simulink model "rx2"  (R2022b)
settings: Solver=FixedStepDiscrete  StartTime=0.0  StopTime=3.3E6  FixedStep=1  RelTol=1e-3  EnableMultiTasking=on
model workspace (MAT data in the model file):
  mwTaskManagerKernelLatency = 0
undefined symbols (not defined in the file or in its folder): Add, jsin, magnitude, rom_pilot_conj_tt, Shift
libraries: hdlsllib x3231, whdlutilities x525, simulink x260, whdlmod x112, whdledac x26, dsphdlmathfun2 x24, commchan3 x1
(part 50 of 59)

== system rx2/process3/decoder/p-p/Subsystem2/Subsystem/Subsystem1/Subsystem/Subsystem4 ==
  data2 : Inport  OutDataTypeStr=data_type
  wr_addr1 : Inport  Port=2
  wr_en2 : Inport  Port=3
  rd_addr1 : Inport  Port=4
  Mux1 : Mux  Inputs=2
  Selector : Selector  InputPortWidth=4  IndexOptions=Index vector (dialog)  Indices=[1:2]  OutputSizes=1
  Selector1 : Selector  InputPortWidth=4  IndexOptions=Index vector (dialog)  Indices=[3:4]  OutputSizes=1
  Subsystem : Subsystem
  Subsystem1 : Subsystem
  rd_dout1 : Outport  PortDimensions=4  VectorParamsAs1DForOutWhenUnconnected=off
  wires:
  Selector/1 -> Subsystem/1(data)
  Subsystem/1(rd_dout) -> Mux1/1
  Subsystem1/1(rd_dout) -> Mux1/2
  wr_addr1/1 -> Subsystem/2(wr_addr), Subsystem1/2(wr_addr)
  Selector1/1 -> Subsystem1/1(data)
  wr_en2/1 -> Subsystem/3(wr_en), Subsystem1/3(wr_en)
  data2/1 -> Selector1/1, Selector/1
  Mux1/1 -> rd_dout1/1
  rd_addr1/1 -> Subsystem/4(rd_addr), Subsystem1/4(rd_addr)

== system rx2/process3/decoder/p-p/Subsystem2/Subsystem/Subsystem1/Subsystem1/Subsystem1 ==
  data2 : Inport  OutDataTypeStr=data_type
  wr_addr1 : Inport  Port=2
  wr_en2 : Inport  Port=3
  rd_addr1 : Inport  Port=4
  Mux1 : Mux  Inputs=2
  Selector : Selector  InputPortWidth=4  IndexOptions=Index vector (dialog)  Indices=[1:2]  OutputSizes=1
  Selector1 : Selector  InputPortWidth=4  IndexOptions=Index vector (dialog)  Indices=[3:4]  OutputSizes=1
  Subsystem : Subsystem
  Subsystem1 : Subsystem
  rd_dout1 : Outport  PortDimensions=4  VectorParamsAs1DForOutWhenUnconnected=off
  wires:
  rd_addr1/1 -> Subsystem1/4(rd_addr), Subsystem/4(rd_addr)
  Mux1/1 -> rd_dout1/1
  data2/1 -> Selector/1, Selector1/1
  wr_en2/1 -> Subsystem1/3(wr_en), Subsystem/3(wr_en)
  Selector1/1 -> Subsystem1/1(data)
  wr_addr1/1 -> Subsystem1/2(wr_addr), Subsystem/2(wr_addr)
  Subsystem1/1(rd_dout) -> Mux1/2
  Subsystem/1(rd_dout) -> Mux1/1
  Selector/1 -> Subsystem/1(data)

== system rx2/process3/decoder/p-p/Subsystem2/Subsystem/Subsystem1/Subsystem1/Subsystem4 ==
  data2 : Inport  OutDataTypeStr=data_type
  wr_addr1 : Inport  Port=2
  wr_en2 : Inport  Port=3
  rd_addr1 : Inport  Port=4
  Mux1 : Mux  Inputs=2
  Selector : Selector  InputPortWidth=4  IndexOptions=Index vector (dialog)  Indices=[1:2]  OutputSizes=1
  Selector1 : Selector  InputPortWidth=4  IndexOptions=Index vector (dialog)  Indices=[3:4]  OutputSizes=1
  Subsystem : Subsystem
  Subsystem1 : Subsystem
  rd_dout1 : Outport  PortDimensions=4  VectorParamsAs1DForOutWhenUnconnected=off
  wires:
  rd_addr1/1 -> Subsystem1/4(rd_addr), Subsystem/4(rd_addr)
  Mux1/1 -> rd_dout1/1
  data2/1 -> Selector/1, Selector1/1
  wr_en2/1 -> Subsystem1/3(wr_en), Subsystem/3(wr_en)
  Selector1/1 -> Subsystem1/1(data)
  wr_addr1/1 -> Subsystem1/2(wr_addr), Subsystem/2(wr_addr)
  Subsystem1/1(rd_dout) -> Mux1/2
  Subsystem/1(rd_dout) -> Mux1/1
  Selector/1 -> Subsystem/1(data)

== system rx2/process3/decoder/p-p/Subsystem2/Subsystem/Subsystem2/Subsystem/Subsystem1 ==
  data2 : Inport  OutDataTypeStr=data_type
  wr_addr1 : Inport  Port=2
  wr_en2 : Inport  Port=3
  rd_addr1 : Inport  Port=4
  Mux1 : Mux  Inputs=2
  Selector : Selector  InputPortWidth=4  IndexOptions=Index vector (dialog)  Indices=[1:2]  OutputSizes=1
  Selector1 : Selector  InputPortWidth=4  IndexOptions=Index vector (dialog)  Indices=[3:4]  OutputSizes=1
  Subsystem : Subsystem
  Subsystem1 : Subsystem
  rd_dout1 : Outport  PortDimensions=4  VectorParamsAs1DForOutWhenUnconnected=off
  wires:
  rd_addr1/1 -> Subsystem1/4(rd_addr), Subsystem/4(rd_addr)
  Mux1/1 -> rd_dout1/1
  data2/1 -> Selector/1, Selector1/1
  wr_en2/1 -> Subsystem1/3(wr_en), Subsystem/3(wr_en)
  Selector1/1 -> Subsystem1/1(data)
  wr_addr1/1 -> Subsystem1/2(wr_addr), Subsystem/2(wr_addr)
  Subsystem1/1(rd_dout) -> Mux1/2
  Subsystem/1(rd_dout) -> Mux1/1
  Selector/1 -> Subsystem/1(data)

== system rx2/process3/decoder/p-p/Subsystem2/Subsystem/Subsystem2/Subsystem/Subsystem4 ==
  data2 : Inport  OutDataTypeStr=data_type
  wr_addr1 : Inport  Port=2
  wr_en2 : Inport  Port=3
  rd_addr1 : Inport  Port=4
  Mux1 : Mux  Inputs=2
  Selector : Selector  InputPortWidth=4  IndexOptions=Index vector (dialog)  Indices=[1:2]  OutputSizes=1
  Selector1 : Selector  InputPortWidth=4  IndexOptions=Index vector (dialog)  Indices=[3:4]  OutputSizes=1
  Subsystem : Subsystem
  Subsystem1 : Subsystem
  rd_dout1 : Outport  PortDimensions=4  VectorParamsAs1DForOutWhenUnconnected=off
  wires:
  Selector/1 -> Subsystem/1(data)
  Subsystem/1(rd_dout) -> Mux1/1
  Subsystem1/1(rd_dout) -> Mux1/2
  wr_addr1/1 -> Subsystem/2(wr_addr), Subsystem1/2(wr_addr)
  Selector1/1 -> Subsystem1/1(data)
  wr_en2/1 -> Subsystem/3(wr_en), Subsystem1/3(wr_en)
  data2/1 -> Selector1/1, Selector/1
  Mux1/1 -> rd_dout1/1
  rd_addr1/1 -> Subsystem/4(rd_addr), Subsystem1/4(rd_addr)

== system rx2/process3/decoder/p-p/Subsystem2/Subsystem/Subsystem2/Subsystem1/Subsystem1 ==
  data2 : Inport  OutDataTypeStr=data_type
  wr_addr1 : Inport  Port=2
  wr_en2 : Inport  Port=3
  rd_addr1 : Inport  Port=4
  Mux1 : Mux  Inputs=2
  Selector : Selector  InputPortWidth=4  IndexOptions=Index vector (dialog)  Indices=[1:2]  OutputSizes=1
  Selector1 : Selector  InputPortWidth=4  IndexOptions=Index vector (dialog)  Indices=[3:4]  OutputSizes=1
  Subsystem : Subsystem
  Subsystem1 : Subsystem
  rd_dout1 : Outport  PortDimensions=4  VectorParamsAs1DForOutWhenUnconnected=off
  wires:
  rd_addr1/1 -> Subsystem1/4(rd_addr), Subsystem/4(rd_addr)
  Mux1/1 -> rd_dout1/1
  data2/1 -> Selector/1, Selector1/1
  wr_en2/1 -> Subsystem1/3(wr_en), Subsystem/3(wr_en)
  Selector1/1 -> Subsystem1/1(data)
  wr_addr1/1 -> Subsystem1/2(wr_addr), Subsystem/2(wr_addr)
  Subsystem1/1(rd_dout) -> Mux1/2
  Subsystem/1(rd_dout) -> Mux1/1
  Selector/1 -> Subsystem/1(data)

== system rx2/process3/decoder/p-p/Subsystem2/Subsystem/Subsystem2/Subsystem1/Subsystem4 ==
  data2 : Inport  OutDataTypeStr=data_type
  wr_addr1 : Inport  Port=2
  wr_en2 : Inport  Port=3
  rd_addr1 : Inport  Port=4
  Mux1 : Mux  Inputs=2
  Selector : Selector  InputPortWidth=4  IndexOptions=Index vector (dialog)  Indices=[1:2]  OutputSizes=1
  Selector1 : Selector  InputPortWidth=4  IndexOptions=Index vector (dialog)  Indices=[3:4]  OutputSizes=1
  Subsystem : Subsystem
  Subsystem1 : Subsystem
  rd_dout1 : Outport  PortDimensions=4  VectorParamsAs1DForOutWhenUnconnected=off
  wires:
  rd_addr1/1 -> Subsystem1/4(rd_addr), Subsystem/4(rd_addr)
  Mux1/1 -> rd_dout1/1
  data2/1 -> Selector/1, Selector1/1
  wr_en2/1 -> Subsystem1/3(wr_en), Subsystem/3(wr_en)
  Selector1/1 -> Subsystem1/1(data)
  wr_addr1/1 -> Subsystem1/2(wr_addr), Subsystem/2(wr_addr)
  Subsystem1/1(rd_dout) -> Mux1/2
  Subsystem/1(rd_dout) -> Mux1/1
  Selector/1 -> Subsystem/1(data)

== system rx2/process3/decoder/p-p/Subsystem2/Subsystem1/Subsystem1/Subsystem/Subsystem1 ==
  data2 : Inport  OutDataTypeStr=data_type
  wr_addr1 : Inport  Port=2
  wr_en2 : Inport  Port=3
  rd_addr1 : Inport  Port=4
  Mux1 : Mux  Inputs=2
  Selector : Selector  InputPortWidth=4  IndexOptions=Index vector (dialog)  Indices=[1:2]  OutputSizes=1
  Selector1 : Selector  InputPortWidth=4  IndexOptions=Index vector (dialog)  Indices=[3:4]  OutputSizes=1
  Subsystem : Subsystem
  Subsystem1 : Subsystem
  rd_dout1 : Outport  PortDimensions=4  VectorParamsAs1DForOutWhenUnconnected=off
  wires:
  rd_addr1/1 -> Subsystem1/4(rd_addr), Subsystem/4(rd_addr)
  Mux1/1 -> rd_dout1/1
  data2/1 -> Selector/1, Selector1/1
  wr_en2/1 -> Subsystem1/3(wr_en), Subsystem/3(wr_en)
  Selector1/1 -> Subsystem1/1(data)
  wr_addr1/1 -> Subsystem1/2(wr_addr), Subsystem/2(wr_addr)
  Subsystem1/1(rd_dout) -> Mux1/2
  Subsystem/1(rd_dout) -> Mux1/1
  Selector/1 -> Subsystem/1(data)

== system rx2/process3/decoder/p-p/Subsystem2/Subsystem1/Subsystem1/Subsystem/Subsystem4 ==
  data2 : Inport  OutDataTypeStr=data_type
  wr_addr1 : Inport  Port=2
  wr_en2 : Inport  Port=3
  rd_addr1 : Inport  Port=4
  Mux1 : Mux  Inputs=2
  Selector : Selector  InputPortWidth=4  IndexOptions=Index vector (dialog)  Indices=[1:2]  OutputSizes=1
  Selector1 : Selector  InputPortWidth=4  IndexOptions=Index vector (dialog)  Indices=[3:4]  OutputSizes=1
  Subsystem : Subsystem
  Subsystem1 : Subsystem
  rd_dout1 : Outport  PortDimensions=4  VectorParamsAs1DForOutWhenUnconnected=off
  wires:
  Selector/1 -> Subsystem/1(data)
  Subsystem/1(rd_dout) -> Mux1/1
  Subsystem1/1(rd_dout) -> Mux1/2
  wr_addr1/1 -> Subsystem/2(wr_addr), Subsystem1/2(wr_addr)
  Selector1/1 -> Subsystem1/1(data)
  wr_en2/1 -> Subsystem/3(wr_en), Subsystem1/3(wr_en)
  data2/1 -> Selector1/1, Selector/1
  Mux1/1 -> rd_dout1/1
  rd_addr1/1 -> Subsystem/4(rd_addr), Subsystem1/4(rd_addr)

== system rx2/process3/decoder/p-p/Subsystem2/Subsystem1/Subsystem1/Subsystem1/Subsystem1 ==
  data2 : Inport  OutDataTypeStr=data_type
  wr_addr1 : Inport  Port=2
  wr_en2 : Inport  Port=3
  rd_addr1 : Inport  Port=4
  Mux1 : Mux  Inputs=2
  Selector : Selector  InputPortWidth=4  IndexOptions=Index vector (dialog)  Indices=[1:2]  OutputSizes=1
  Selector1 : Selector  InputPortWidth=4  IndexOptions=Index vector (dialog)  Indices=[3:4]  OutputSizes=1
  Subsystem : Subsystem
  Subsystem1 : Subsystem
  rd_dout1 : Outport  PortDimensions=4  VectorParamsAs1DForOutWhenUnconnected=off
  wires:
  rd_addr1/1 -> Subsystem1/4(rd_addr), Subsystem/4(rd_addr)
  Mux1/1 -> rd_dout1/1
  data2/1 -> Selector/1, Selector1/1
  wr_en2/1 -> Subsystem1/3(wr_en), Subsystem/3(wr_en)
  Selector1/1 -> Subsystem1/1(data)
  wr_addr1/1 -> Subsystem1/2(wr_addr), Subsystem/2(wr_addr)
  Subsystem1/1(rd_dout) -> Mux1/2
  Subsystem/1(rd_dout) -> Mux1/1
  Selector/1 -> Subsystem/1(data)

== system rx2/process3/decoder/p-p/Subsystem2/Subsystem1/Subsystem1/Subsystem1/Subsystem4 ==
  data2 : Inport  OutDataTypeStr=data_type
  wr_addr1 : Inport  Port=2
  wr_en2 : Inport  Port=3
  rd_addr1 : Inport  Port=4
  Mux1 : Mux  Inputs=2
  Selector : Selector  InputPortWidth=4  IndexOptions=Index vector (dialog)  Indices=[1:2]  OutputSizes=1
  Selector1 : Selector  InputPortWidth=4  IndexOptions=Index vector (dialog)  Indices=[3:4]  OutputSizes=1
  Subsystem : Subsystem
  Subsystem1 : Subsystem
  rd_dout1 : Outport  PortDimensions=4  VectorParamsAs1DForOutWhenUnconnected=off
  wires:
  rd_addr1/1 -> Subsystem1/4(rd_addr), Subsystem/4(rd_addr)
  Mux1/1 -> rd_dout1/1
  data2/1 -> Selector/1, Selector1/1
  wr_en2/1 -> Subsystem1/3(wr_en), Subsystem/3(wr_en)
  Selector1/1 -> Subsystem1/1(data)
  wr_addr1/1 -> Subsystem1/2(wr_addr), Subsystem/2(wr_addr)
  Subsystem1/1(rd_dout) -> Mux1/2
  Subsystem/1(rd_dout) -> Mux1/1
  Selector/1 -> Subsystem/1(data)

== system rx2/process3/decoder/p-p/Subsystem2/Subsystem1/Subsystem2/Subsystem/Subsystem1 ==
  data2 : Inport  OutDataTypeStr=data_type
  wr_addr1 : Inport  Port=2
  wr_en2 : Inport  Port=3
  rd_addr1 : Inport  Port=4
  Mux1 : Mux  Inputs=2
  Selector : Selector  InputPortWidth=4  IndexOptions=Index vector (dialog)  Indices=[1:2]  OutputSizes=1
  Selector1 : Selector  InputPortWidth=4  IndexOptions=Index vector (dialog)  Indices=[3:4]  OutputSizes=1
  Subsystem : Subsystem
  Subsystem1 : Subsystem
  rd_dout1 : Outport  PortDimensions=4  VectorParamsAs1DForOutWhenUnconnected=off
  wires:
  rd_addr1/1 -> Subsystem1/4(rd_addr), Subsystem/4(rd_addr)
  Mux1/1 -> rd_dout1/1
  data2/1 -> Selector/1, Selector1/1
  wr_en2/1 -> Subsystem1/3(wr_en), Subsystem/3(wr_en)
  Selector1/1 -> Subsystem1/1(data)
  wr_addr1/1 -> Subsystem1/2(wr_addr), Subsystem/2(wr_addr)
  Subsystem1/1(rd_dout) -> Mux1/2
  Subsystem/1(rd_dout) -> Mux1/1
  Selector/1 -> Subsystem/1(data)

== system rx2/process3/decoder/p-p/Subsystem2/Subsystem1/Subsystem2/Subsystem/Subsystem4 ==
  data2 : Inport  OutDataTypeStr=data_type
  wr_addr1 : Inport  Port=2
  wr_en2 : Inport  Port=3
  rd_addr1 : Inport  Port=4
  Mux1 : Mux  Inputs=2
  Selector : Selector  InputPortWidth=4  IndexOptions=Index vector (dialog)  Indices=[1:2]  OutputSizes=1
  Selector1 : Selector  InputPortWidth=4  IndexOptions=Index vector (dialog)  Indices=[3:4]  OutputSizes=1
  Subsystem : Subsystem
  Subsystem1 : Subsystem
  rd_dout1 : Outport  PortDimensions=4  VectorParamsAs1DForOutWhenUnconnected=off
  wires:
  Selector/1 -> Subsystem/1(data)
  Subsystem/1(rd_dout) -> Mux1/1
  Subsystem1/1(rd_dout) -> Mux1/2
  wr_addr1/1 -> Subsystem/2(wr_addr), Subsystem1/2(wr_addr)
  Selector1/1 -> Subsystem1/1(data)
  wr_en2/1 -> Subsystem/3(wr_en), Subsystem1/3(wr_en)
  data2/1 -> Selector1/1, Selector/1
  Mux1/1 -> rd_dout1/1
  rd_addr1/1 -> Subsystem/4(rd_addr), Subsystem1/4(rd_addr)

== system rx2/process3/decoder/p-p/Subsystem2/Subsystem1/Subsystem2/Subsystem1/Subsystem1 ==
  data2 : Inport  OutDataTypeStr=data_type
  wr_addr1 : Inport  Port=2
  wr_en2 : Inport  Port=3
  rd_addr1 : Inport  Port=4
  Mux1 : Mux  Inputs=2
  Selector : Selector  InputPortWidth=4  IndexOptions=Index vector (dialog)  Indices=[1:2]  OutputSizes=1
  Selector1 : Selector  InputPortWidth=4  IndexOptions=Index vector (dialog)  Indices=[3:4]  OutputSizes=1
  Subsystem : Subsystem
  Subsystem1 : Subsystem
  rd_dout1 : Outport  PortDimensions=4  VectorParamsAs1DForOutWhenUnconnected=off
  wires:
  rd_addr1/1 -> Subsystem1/4(rd_addr), Subsystem/4(rd_addr)
  Mux1/1 -> rd_dout1/1
  data2/1 -> Selector/1, Selector1/1
  wr_en2/1 -> Subsystem1/3(wr_en), Subsystem/3(wr_en)
  Selector1/1 -> Subsystem1/1(data)
  wr_addr1/1 -> Subsystem1/2(wr_addr), Subsystem/2(wr_addr)
  Subsystem1/1(rd_dout) -> Mux1/2
  Subsystem/1(rd_dout) -> Mux1/1
  Selector/1 -> Subsystem/1(data)

== system rx2/process3/decoder/p-p/Subsystem2/Subsystem1/Subsystem2/Subsystem1/Subsystem4 ==
  data2 : Inport  OutDataTypeStr=data_type
  wr_addr1 : Inport  Port=2
  wr_en2 : Inport  Port=3
  rd_addr1 : Inport  Port=4
  Mux1 : Mux  Inputs=2
  Selector : Selector  InputPortWidth=4  IndexOptions=Index vector (dialog)  Indices=[1:2]  OutputSizes=1
  Selector1 : Selector  InputPortWidth=4  IndexOptions=Index vector (dialog)  Indices=[3:4]  OutputSizes=1
  Subsystem : Subsystem
  Subsystem1 : Subsystem
  rd_dout1 : Outport  PortDimensions=4  VectorParamsAs1DForOutWhenUnconnected=off
  wires:
  rd_addr1/1 -> Subsystem1/4(rd_addr), Subsystem/4(rd_addr)
  Mux1/1 -> rd_dout1/1
  data2/1 -> Selector/1, Selector1/1
  wr_en2/1 -> Subsystem1/3(wr_en), Subsystem/3(wr_en)
  Selector1/1 -> Subsystem1/1(data)
  wr_addr1/1 -> Subsystem1/2(wr_addr), Subsystem/2(wr_addr)
  Subsystem1/1(rd_dout) -> Mux1/2
  Subsystem/1(rd_dout) -> Mux1/1
  Selector/1 -> Subsystem/1(data)

== system rx2/process4/decoder/p-p/Subsystem2/Subsystem/Subsystem1/Subsystem/Subsystem1 ==
  data2 : Inport  OutDataTypeStr=data_type
  wr_addr1 : Inport  Port=2
  wr_en2 : Inport  Port=3
  rd_addr1 : Inport  Port=4
  Mux1 : Mux  Inputs=2
  Selector : Selector  InputPortWidth=4  IndexOptions=Index vector (dialog)  Indices=[1:2]  OutputSizes=1
  Selector1 : Selector  InputPortWidth=4  IndexOptions=Index vector (dialog)  Indices=[3:4]  OutputSizes=1
  Subsystem : Subsystem
  Subsystem1 : Subsystem
  rd_dout1 : Outport  PortDimensions=4  VectorParamsAs1DForOutWhenUnconnected=off
  wires:
  Selector/1 -> Subsystem/1(data)
  Subsystem/1(rd_dout) -> Mux1/1
  Subsystem1/1(rd_dout) -> Mux1/2
  wr_addr1/1 -> Subsystem/2(wr_addr), Subsystem1/2(wr_addr)
  Selector1/1 -> Subsystem1/1(data)
  wr_en2/1 -> Subsystem/3(wr_en), Subsystem1/3(wr_en)
  data2/1 -> Selector1/1, Selector/1
  Mux1/1 -> rd_dout1/1
  rd_addr1/1 -> Subsystem/4(rd_addr), Subsystem1/4(rd_addr)

== system rx2/process4/decoder/p-p/Subsystem2/Subsystem/Subsystem1/Subsystem/Subsystem4 ==
  data2 : Inport  OutDataTypeStr=data_type
  wr_addr1 : Inport  Port=2
  wr_en2 : Inport  Port=3
  rd_addr1 : Inport  Port=4
  Mux1 : Mux  Inputs=2
  Selector : Selector  InputPortWidth=4  IndexOptions=Index vector (dialog)  Indices=[1:2]  OutputSizes=1
  Selector1 : Selector  InputPortWidth=4  IndexOptions=Index vector (dialog)  Indices=[3:4]  OutputSizes=1
  Subsystem : Subsystem
  Subsystem1 : Subsystem
  rd_dout1 : Outport  PortDimensions=4  VectorParamsAs1DForOutWhenUnconnected=off
  wires:
  rd_addr1/1 -> Subsystem1/4(rd_addr), Subsystem/4(rd_addr)
  Mux1/1 -> rd_dout1/1
  data2/1 -> Selector/1, Selector1/1
  wr_en2/1 -> Subsystem1/3(wr_en), Subsystem/3(wr_en)
  Selector1/1 -> Subsystem1/1(data)
  wr_addr1/1 -> Subsystem1/2(wr_addr), Subsystem/2(wr_addr)
  Subsystem1/1(rd_dout) -> Mux1/2
  Subsystem/1(rd_dout) -> Mux1/1
  Selector/1 -> Subsystem/1(data)

== system rx2/process4/decoder/p-p/Subsystem2/Subsystem/Subsystem1/Subsystem1/Subsystem1 ==
  data2 : Inport  OutDataTypeStr=data_type
  wr_addr1 : Inport  Port=2
  wr_en2 : Inport  Port=3
  rd_addr1 : Inport  Port=4
  Mux1 : Mux  Inputs=2
  Selector : Selector  InputPortWidth=4  IndexOptions=Index vector (dialog)  Indices=[1:2]  OutputSizes=1
  Selector1 : Selector  InputPortWidth=4  IndexOptions=Index vector (dialog)  Indices=[3:4]  OutputSizes=1
  Subsystem : Subsystem
  Subsystem1 : Subsystem
  rd_dout1 : Outport  PortDimensions=4  VectorParamsAs1DForOutWhenUnconnected=off
  wires:
  Selector/1 -> Subsystem/1(data)
  Subsystem/1(rd_dout) -> Mux1/1
  Subsystem1/1(rd_dout) -> Mux1/2
  wr_addr1/1 -> Subsystem/2(wr_addr), Subsystem1/2(wr_addr)
  Selector1/1 -> Subsystem1/1(data)
  wr_en2/1 -> Subsystem/3(wr_en), Subsystem1/3(wr_en)
  data2/1 -> Selector1/1, Selector/1
  Mux1/1 -> rd_dout1/1
  rd_addr1/1 -> Subsystem/4(rd_addr), Subsystem1/4(rd_addr)

== system rx2/process4/decoder/p-p/Subsystem2/Subsystem/Subsystem1/Subsystem1/Subsystem4 ==
  data2 : Inport  OutDataTypeStr=data_type
  wr_addr1 : Inport  Port=2
  wr_en2 : Inport  Port=3
  rd_addr1 : Inport  Port=4
  Mux1 : Mux  Inputs=2
  Selector : Selector  InputPortWidth=4  IndexOptions=Index vector (dialog)  Indices=[1:2]  OutputSizes=1
  Selector1 : Selector  InputPortWidth=4  IndexOptions=Index vector (dialog)  Indices=[3:4]  OutputSizes=1
  Subsystem : Subsystem
  Subsystem1 : Subsystem
  rd_dout1 : Outport  PortDimensions=4  VectorParamsAs1DForOutWhenUnconnected=off
  wires:
  Selector/1 -> Subsystem/1(data)
  Subsystem/1(rd_dout) -> Mux1/1
  Subsystem1/1(rd_dout) -> Mux1/2
  wr_addr1/1 -> Subsystem/2(wr_addr), Subsystem1/2(wr_addr)
  Selector1/1 -> Subsystem1/1(data)
  wr_en2/1 -> Subsystem/3(wr_en), Subsystem1/3(wr_en)
  data2/1 -> Selector1/1, Selector/1
  Mux1/1 -> rd_dout1/1
  rd_addr1/1 -> Subsystem/4(rd_addr), Subsystem1/4(rd_addr)

== system rx2/process4/decoder/p-p/Subsystem2/Subsystem/Subsystem2/Subsystem/Subsystem1 ==
  data2 : Inport  OutDataTypeStr=data_type
  wr_addr1 : Inport  Port=2
  wr_en2 : Inport  Port=3
  rd_addr1 : Inport  Port=4
  Mux1 : Mux  Inputs=2
  Selector : Selector  InputPortWidth=4  IndexOptions=Index vector (dialog)  Indices=[1:2]  OutputSizes=1
  Selector1 : Selector  InputPortWidth=4  IndexOptions=Index vector (dialog)  Indices=[3:4]  OutputSizes=1
  Subsystem : Subsystem
  Subsystem1 : Subsystem
  rd_dout1 : Outport  PortDimensions=4  VectorParamsAs1DForOutWhenUnconnected=off
  wires:
  Selector/1 -> Subsystem/1(data)
  Subsystem/1(rd_dout) -> Mux1/1
  Subsystem1/1(rd_dout) -> Mux1/2
  wr_addr1/1 -> Subsystem/2(wr_addr), Subsystem1/2(wr_addr)
  Selector1/1 -> Subsystem1/1(data)
  wr_en2/1 -> Subsystem/3(wr_en), Subsystem1/3(wr_en)
  data2/1 -> Selector1/1, Selector/1
  Mux1/1 -> rd_dout1/1
  rd_addr1/1 -> Subsystem/4(rd_addr), Subsystem1/4(rd_addr)

== system rx2/process4/decoder/p-p/Subsystem2/Subsystem/Subsystem2/Subsystem/Subsystem4 ==
  data2 : Inport  OutDataTypeStr=data_type
  wr_addr1 : Inport  Port=2
  wr_en2 : Inport  Port=3
  rd_addr1 : Inport  Port=4
  Mux1 : Mux  Inputs=2
  Selector : Selector  InputPortWidth=4  IndexOptions=Index vector (dialog)  Indices=[1:2]  OutputSizes=1
  Selector1 : Selector  InputPortWidth=4  IndexOptions=Index vector (dialog)  Indices=[3:4]  OutputSizes=1
  Subsystem : Subsystem
  Subsystem1 : Subsystem
  rd_dout1 : Outport  PortDimensions=4  VectorParamsAs1DForOutWhenUnconnected=off
  wires:
  rd_addr1/1 -> Subsystem1/4(rd_addr), Subsystem/4(rd_addr)
  Mux1/1 -> rd_dout1/1
  data2/1 -> Selector/1, Selector1/1
  wr_en2/1 -> Subsystem1/3(wr_en), Subsystem/3(wr_en)
  Selector1/1 -> Subsystem1/1(data)
  wr_addr1/1 -> Subsystem1/2(wr_addr), Subsystem/2(wr_addr)
  Subsystem1/1(rd_dout) -> Mux1/2
  Subsystem/1(rd_dout) -> Mux1/1
  Selector/1 -> Subsystem/1(data)

== system rx2/process4/decoder/p-p/Subsystem2/Subsystem/Subsystem2/Subsystem1/Subsystem1 ==
  data2 : Inport  OutDataTypeStr=data_type
  wr_addr1 : Inport  Port=2
  wr_en2 : Inport  Port=3
  rd_addr1 : Inport  Port=4
  Mux1 : Mux  Inputs=2
  Selector : Selector  InputPortWidth=4  IndexOptions=Index vector (dialog)  Indices=[1:2]  OutputSizes=1
  Selector1 : Selector  InputPortWidth=4  IndexOptions=Index vector (dialog)  Indices=[3:4]  OutputSizes=1
  Subsystem : Subsystem
  Subsystem1 : Subsystem
  rd_dout1 : Outport  PortDimensions=4  VectorParamsAs1DForOutWhenUnconnected=off
  wires:
  Selector/1 -> Subsystem/1(data)
  Subsystem/1(rd_dout) -> Mux1/1
  Subsystem1/1(rd_dout) -> Mux1/2
  wr_addr1/1 -> Subsystem/2(wr_addr), Subsystem1/2(wr_addr)
  Selector1/1 -> Subsystem1/1(data)
  wr_en2/1 -> Subsystem/3(wr_en), Subsystem1/3(wr_en)
  data2/1 -> Selector1/1, Selector/1
  Mux1/1 -> rd_dout1/1
  rd_addr1/1 -> Subsystem/4(rd_addr), Subsystem1/4(rd_addr)

== system rx2/process4/decoder/p-p/Subsystem2/Subsystem/Subsystem2/Subsystem1/Subsystem4 ==
  data2 : Inport  OutDataTypeStr=data_type
  wr_addr1 : Inport  Port=2
  wr_en2 : Inport  Port=3
  rd_addr1 : Inport  Port=4
  Mux1 : Mux  Inputs=2
  Selector : Selector  InputPortWidth=4  IndexOptions=Index vector (dialog)  Indices=[1:2]  OutputSizes=1
  Selector1 : Selector  InputPortWidth=4  IndexOptions=Index vector (dialog)  Indices=[3:4]  OutputSizes=1
  Subsystem : Subsystem
  Subsystem1 : Subsystem
  rd_dout1 : Outport  PortDimensions=4  VectorParamsAs1DForOutWhenUnconnected=off
  wires:
  Selector/1 -> Subsystem/1(data)
  Subsystem/1(rd_dout) -> Mux1/1
  Subsystem1/1(rd_dout) -> Mux1/2
  wr_addr1/1 -> Subsystem/2(wr_addr), Subsystem1/2(wr_addr)
  Selector1/1 -> Subsystem1/1(data)
  wr_en2/1 -> Subsystem/3(wr_en), Subsystem1/3(wr_en)
  data2/1 -> Selector1/1, Selector/1
  Mux1/1 -> rd_dout1/1
  rd_addr1/1 -> Subsystem/4(rd_addr), Subsystem1/4(rd_addr)

== system rx2/process4/decoder/p-p/Subsystem2/Subsystem1/Subsystem1/Subsystem/Subsystem1 ==
  data2 : Inport  OutDataTypeStr=data_type
  wr_addr1 : Inport  Port=2
  wr_en2 : Inport  Port=3
  rd_addr1 : Inport  Port=4
  Mux1 : Mux  Inputs=2
  Selector : Selector  InputPortWidth=4  IndexOptions=Index vector (dialog)  Indices=[1:2]  OutputSizes=1
  Selector1 : Selector  InputPortWidth=4  IndexOptions=Index vector (dialog)  Indices=[3:4]  OutputSizes=1
  Subsystem : Subsystem
  Subsystem1 : Subsystem
  rd_dout1 : Outport  PortDimensions=4  VectorParamsAs1DForOutWhenUnconnected=off
  wires:
  Selector/1 -> Subsystem/1(data)
  Subsystem/1(rd_dout) -> Mux1/1
  Subsystem1/1(rd_dout) -> Mux1/2
  wr_addr1/1 -> Subsystem/2(wr_addr), Subsystem1/2(wr_addr)
  Selector1/1 -> Subsystem1/1(data)
  wr_en2/1 -> Subsystem/3(wr_en), Subsystem1/3(wr_en)
  data2/1 -> Selector1/1, Selector/1
  Mux1/1 -> rd_dout1/1
  rd_addr1/1 -> Subsystem/4(rd_addr), Subsystem1/4(rd_addr)

== system rx2/process4/decoder/p-p/Subsystem2/Subsystem1/Subsystem1/Subsystem/Subsystem4 ==
  data2 : Inport  OutDataTypeStr=data_type
  wr_addr1 : Inport  Port=2
  wr_en2 : Inport  Port=3
  rd_addr1 : Inport  Port=4
  Mux1 : Mux  Inputs=2
  Selector : Selector  InputPortWidth=4  IndexOptions=Index vector (dialog)  Indices=[1:2]  OutputSizes=1
  Selector1 : Selector  InputPortWidth=4  IndexOptions=Index vector (dialog)  Indices=[3:4]  OutputSizes=1
  Subsystem : Subsystem
  Subsystem1 : Subsystem
  rd_dout1 : Outport  PortDimensions=4  VectorParamsAs1DForOutWhenUnconnected=off
  wires:
  rd_addr1/1 -> Subsystem1/4(rd_addr), Subsystem/4(rd_addr)
  Mux1/1 -> rd_dout1/1
  data2/1 -> Selector/1, Selector1/1
  wr_en2/1 -> Subsystem1/3(wr_en), Subsystem/3(wr_en)
  Selector1/1 -> Subsystem1/1(data)
  wr_addr1/1 -> Subsystem1/2(wr_addr), Subsystem/2(wr_addr)
  Subsystem1/1(rd_dout) -> Mux1/2
  Subsystem/1(rd_dout) -> Mux1/1
  Selector/1 -> Subsystem/1(data)

== system rx2/process4/decoder/p-p/Subsystem2/Subsystem1/Subsystem1/Subsystem1/Subsystem1 ==
  data2 : Inport  OutDataTypeStr=data_type
  wr_addr1 : Inport  Port=2
  wr_en2 : Inport  Port=3
  rd_addr1 : Inport  Port=4
  Mux1 : Mux  Inputs=2
  Selector : Selector  InputPortWidth=4  IndexOptions=Index vector (dialog)  Indices=[1:2]  OutputSizes=1
  Selector1 : Selector  InputPortWidth=4  IndexOptions=Index vector (dialog)  Indices=[3:4]  OutputSizes=1
  Subsystem : Subsystem
  Subsystem1 : Subsystem
  rd_dout1 : Outport  PortDimensions=4  VectorParamsAs1DForOutWhenUnconnected=off
  wires:
  Selector/1 -> Subsystem/1(data)
  Subsystem/1(rd_dout) -> Mux1/1
  Subsystem1/1(rd_dout) -> Mux1/2
  wr_addr1/1 -> Subsystem/2(wr_addr), Subsystem1/2(wr_addr)
  Selector1/1 -> Subsystem1/1(data)
  wr_en2/1 -> Subsystem/3(wr_en), Subsystem1/3(wr_en)
  data2/1 -> Selector1/1, Selector/1
  Mux1/1 -> rd_dout1/1
  rd_addr1/1 -> Subsystem/4(rd_addr), Subsystem1/4(rd_addr)

== system rx2/process4/decoder/p-p/Subsystem2/Subsystem1/Subsystem1/Subsystem1/Subsystem4 ==
  data2 : Inport  OutDataTypeStr=data_type
  wr_addr1 : Inport  Port=2
  wr_en2 : Inport  Port=3
  rd_addr1 : Inport  Port=4
  Mux1 : Mux  Inputs=2
  Selector : Selector  InputPortWidth=4  IndexOptions=Index vector (dialog)  Indices=[1:2]  OutputSizes=1
  Selector1 : Selector  InputPortWidth=4  IndexOptions=Index vector (dialog)  Indices=[3:4]  OutputSizes=1
  Subsystem : Subsystem
  Subsystem1 : Subsystem
  rd_dout1 : Outport  PortDimensions=4  VectorParamsAs1DForOutWhenUnconnected=off
  wires:
  Selector/1 -> Subsystem/1(data)
  Subsystem/1(rd_dout) -> Mux1/1
  Subsystem1/1(rd_dout) -> Mux1/2
  wr_addr1/1 -> Subsystem/2(wr_addr), Subsystem1/2(wr_addr)
  Selector1/1 -> Subsystem1/1(data)
  wr_en2/1 -> Subsystem/3(wr_en), Subsystem1/3(wr_en)
  data2/1 -> Selector1/1, Selector/1
  Mux1/1 -> rd_dout1/1
  rd_addr1/1 -> Subsystem/4(rd_addr), Subsystem1/4(rd_addr)

== system rx2/process4/decoder/p-p/Subsystem2/Subsystem1/Subsystem2/Subsystem/Subsystem1 ==
  data2 : Inport  OutDataTypeStr=data_type
  wr_addr1 : Inport  Port=2
  wr_en2 : Inport  Port=3
  rd_addr1 : Inport  Port=4
  Mux1 : Mux  Inputs=2
  Selector : Selector  InputPortWidth=4  IndexOptions=Index vector (dialog)  Indices=[1:2]  OutputSizes=1
  Selector1 : Selector  InputPortWidth=4  IndexOptions=Index vector (dialog)  Indices=[3:4]  OutputSizes=1
  Subsystem : Subsystem
  Subsystem1 : Subsystem
  rd_dout1 : Outport  PortDimensions=4  VectorParamsAs1DForOutWhenUnconnected=off
  wires:
  Selector/1 -> Subsystem/1(data)
  Subsystem/1(rd_dout) -> Mux1/1
  Subsystem1/1(rd_dout) -> Mux1/2
  wr_addr1/1 -> Subsystem/2(wr_addr), Subsystem1/2(wr_addr)
  Selector1/1 -> Subsystem1/1(data)
  wr_en2/1 -> Subsystem/3(wr_en), Subsystem1/3(wr_en)
  data2/1 -> Selector1/1, Selector/1
  Mux1/1 -> rd_dout1/1
  rd_addr1/1 -> Subsystem/4(rd_addr), Subsystem1/4(rd_addr)

== system rx2/process4/decoder/p-p/Subsystem2/Subsystem1/Subsystem2/Subsystem/Subsystem4 ==
  data2 : Inport  OutDataTypeStr=data_type
  wr_addr1 : Inport  Port=2
  wr_en2 : Inport  Port=3
  rd_addr1 : Inport  Port=4
  Mux1 : Mux  Inputs=2
  Selector : Selector  InputPortWidth=4  IndexOptions=Index vector (dialog)  Indices=[1:2]  OutputSizes=1
  Selector1 : Selector  InputPortWidth=4  IndexOptions=Index vector (dialog)  Indices=[3:4]  OutputSizes=1
  Subsystem : Subsystem
  Subsystem1 : Subsystem
  rd_dout1 : Outport  PortDimensions=4  VectorParamsAs1DForOutWhenUnconnected=off
  wires:
  rd_addr1/1 -> Subsystem1/4(rd_addr), Subsystem/4(rd_addr)
  Mux1/1 -> rd_dout1/1
  data2/1 -> Selector/1, Selector1/1
  wr_en2/1 -> Subsystem1/3(wr_en), Subsystem/3(wr_en)
  Selector1/1 -> Subsystem1/1(data)
  wr_addr1/1 -> Subsystem1/2(wr_addr), Subsystem/2(wr_addr)
  Subsystem1/1(rd_dout) -> Mux1/2
  Subsystem/1(rd_dout) -> Mux1/1
  Selector/1 -> Subsystem/1(data)

== system rx2/process4/decoder/p-p/Subsystem2/Subsystem1/Subsystem2/Subsystem1/Subsystem1 ==
  data2 : Inport  OutDataTypeStr=data_type
  wr_addr1 : Inport  Port=2
  wr_en2 : Inport  Port=3
  rd_addr1 : Inport  Port=4
  Mux1 : Mux  Inputs=2
  Selector : Selector  InputPortWidth=4  IndexOptions=Index vector (dialog)  Indices=[1:2]  OutputSizes=1
  Selector1 : Selector  InputPortWidth=4  IndexOptions=Index vector (dialog)  Indices=[3:4]  OutputSizes=1
  Subsystem : Subsystem
  Subsystem1 : Subsystem
  rd_dout1 : Outport  PortDimensions=4  VectorParamsAs1DForOutWhenUnconnected=off
  wires:
  Selector/1 -> Subsystem/1(data)
  Subsystem/1(rd_dout) -> Mux1/1
  Subsystem1/1(rd_dout) -> Mux1/2
  wr_addr1/1 -> Subsystem/2(wr_addr), Subsystem1/2(wr_addr)
  Selector1/1 -> Subsystem1/1(data)
  wr_en2/1 -> Subsystem/3(wr_en), Subsystem1/3(wr_en)
  data2/1 -> Selector1/1, Selector/1
  Mux1/1 -> rd_dout1/1
  rd_addr1/1 -> Subsystem/4(rd_addr), Subsystem1/4(rd_addr)

== system rx2/process4/decoder/p-p/Subsystem2/Subsystem1/Subsystem2/Subsystem1/Subsystem4 ==
  data2 : Inport  OutDataTypeStr=data_type
  wr_addr1 : Inport  Port=2
  wr_en2 : Inport  Port=3
  rd_addr1 : Inport  Port=4
  Mux1 : Mux  Inputs=2
  Selector : Selector  InputPortWidth=4  IndexOptions=Index vector (dialog)  Indices=[1:2]  OutputSizes=1
  Selector1 : Selector  InputPortWidth=4  IndexOptions=Index vector (dialog)  Indices=[3:4]  OutputSizes=1
  Subsystem : Subsystem
  Subsystem1 : Subsystem
  rd_dout1 : Outport  PortDimensions=4  VectorParamsAs1DForOutWhenUnconnected=off
  wires:
  Selector/1 -> Subsystem/1(data)
  Subsystem/1(rd_dout) -> Mux1/1
  Subsystem1/1(rd_dout) -> Mux1/2
  wr_addr1/1 -> Subsystem/2(wr_addr), Subsystem1/2(wr_addr)
  Selector1/1 -> Subsystem1/1(data)
  wr_en2/1 -> Subsystem/3(wr_en), Subsystem1/3(wr_en)
  data2/1 -> Selector1/1, Selector/1
  Mux1/1 -> rd_dout1/1
  rd_addr1/1 -> Subsystem/4(rd_addr), Subsystem1/4(rd_addr)

== system rx2/process5/decoder/p-p/Subsystem2/Subsystem/Subsystem1/Subsystem/Subsystem1 ==
  data2 : Inport  OutDataTypeStr=data_type
  wr_addr1 : Inport  Port=2
  wr_en2 : Inport  Port=3
  rd_addr1 : Inport  Port=4
  Mux1 : Mux  Inputs=2
  Selector : Selector  InputPortWidth=4  IndexOptions=Index vector (dialog)  Indices=[1:2]  OutputSizes=1
  Selector1 : Selector  InputPortWidth=4  IndexOptions=Index vector (dialog)  Indices=[3:4]  OutputSizes=1
  Subsystem : Subsystem
  Subsystem1 : Subsystem
  rd_dout1 : Outport  PortDimensions=4  VectorParamsAs1DForOutWhenUnconnected=off
  wires:
  rd_addr1/1 -> Subsystem1/4(rd_addr), Subsystem/4(rd_addr)
  Mux1/1 -> rd_dout1/1
  data2/1 -> Selector/1, Selector1/1
  wr_en2/1 -> Subsystem1/3(wr_en), Subsystem/3(wr_en)
  Selector1/1 -> Subsystem1/1(data)
  wr_addr1/1 -> Subsystem1/2(wr_addr), Subsystem/2(wr_addr)
  Subsystem1/1(rd_dout) -> Mux1/2
  Subsystem/1(rd_dout) -> Mux1/1
  Selector/1 -> Subsystem/1(data)

== system rx2/process5/decoder/p-p/Subsystem2/Subsystem/Subsystem1/Subsystem/Subsystem4 ==
  data2 : Inport  OutDataTypeStr=data_type
  wr_addr1 : Inport  Port=2
  wr_en2 : Inport  Port=3
  rd_addr1 : Inport  Port=4
  Mux1 : Mux  Inputs=2
  Selector : Selector  InputPortWidth=4  IndexOptions=Index vector (dialog)  Indices=[1:2]  OutputSizes=1
  Selector1 : Selector  InputPortWidth=4  IndexOptions=Index vector (dialog)  Indices=[3:4]  OutputSizes=1
  Subsystem : Subsystem
  Subsystem1 : Subsystem
  rd_dout1 : Outport  PortDimensions=4  VectorParamsAs1DForOutWhenUnconnected=off
  wires:
  Selector/1 -> Subsystem/1(data)
  Subsystem/1(rd_dout) -> Mux1/1
  Subsystem1/1(rd_dout) -> Mux1/2
  wr_addr1/1 -> Subsystem/2(wr_addr), Subsystem1/2(wr_addr)
  Selector1/1 -> Subsystem1/1(data)
  wr_en2/1 -> Subsystem/3(wr_en), Subsystem1/3(wr_en)
  data2/1 -> Selector1/1, Selector/1
  Mux1/1 -> rd_dout1/1
  rd_addr1/1 -> Subsystem/4(rd_addr), Subsystem1/4(rd_addr)

== system rx2/process5/decoder/p-p/Subsystem2/Subsystem/Subsystem1/Subsystem1/Subsystem1 ==
  data2 : Inport  OutDataTypeStr=data_type
  wr_addr1 : Inport  Port=2
  wr_en2 : Inport  Port=3
  rd_addr1 : Inport  Port=4
  Mux1 : Mux  Inputs=2
  Selector : Selector  InputPortWidth=4  IndexOptions=Index vector (dialog)  Indices=[1:2]  OutputSizes=1
  Selector1 : Selector  InputPortWidth=4  IndexOptions=Index vector (dialog)  Indices=[3:4]  OutputSizes=1
  Subsystem : Subsystem
  Subsystem1 : Subsystem
  rd_dout1 : Outport  PortDimensions=4  VectorParamsAs1DForOutWhenUnconnected=off
  wires:
  rd_addr1/1 -> Subsystem1/4(rd_addr), Subsystem/4(rd_addr)
  Mux1/1 -> rd_dout1/1
  data2/1 -> Selector/1, Selector1/1
  wr_en2/1 -> Subsystem1/3(wr_en), Subsystem/3(wr_en)
  Selector1/1 -> Subsystem1/1(data)
  wr_addr1/1 -> Subsystem1/2(wr_addr), Subsystem/2(wr_addr)
  Subsystem1/1(rd_dout) -> Mux1/2
  Subsystem/1(rd_dout) -> Mux1/1
  Selector/1 -> Subsystem/1(data)

== system rx2/process5/decoder/p-p/Subsystem2/Subsystem/Subsystem1/Subsystem1/Subsystem4 ==
  data2 : Inport  OutDataTypeStr=data_type
  wr_addr1 : Inport  Port=2
  wr_en2 : Inport  Port=3
  rd_addr1 : Inport  Port=4
  Mux1 : Mux  Inputs=2
  Selector : Selector  InputPortWidth=4  IndexOptions=Index vector (dialog)  Indices=[1:2]  OutputSizes=1
  Selector1 : Selector  InputPortWidth=4  IndexOptions=Index vector (dialog)  Indices=[3:4]  OutputSizes=1
  Subsystem : Subsystem
  Subsystem1 : Subsystem
  rd_dout1 : Outport  PortDimensions=4  VectorParamsAs1DForOutWhenUnconnected=off
  wires:
  rd_addr1/1 -> Subsystem1/4(rd_addr), Subsystem/4(rd_addr)
  Mux1/1 -> rd_dout1/1
  data2/1 -> Selector/1, Selector1/1
  wr_en2/1 -> Subsystem1/3(wr_en), Subsystem/3(wr_en)
  Selector1/1 -> Subsystem1/1(data)
  wr_addr1/1 -> Subsystem1/2(wr_addr), Subsystem/2(wr_addr)
  Subsystem1/1(rd_dout) -> Mux1/2
  Subsystem/1(rd_dout) -> Mux1/1
  Selector/1 -> Subsystem/1(data)

== system rx2/process5/decoder/p-p/Subsystem2/Subsystem/Subsystem2/Subsystem/Subsystem1 ==
  data2 : Inport  OutDataTypeStr=data_type
  wr_addr1 : Inport  Port=2
  wr_en2 : Inport  Port=3
  rd_addr1 : Inport  Port=4
  Mux1 : Mux  Inputs=2
  Selector : Selector  InputPortWidth=4  IndexOptions=Index vector (dialog)  Indices=[1:2]  OutputSizes=1
  Selector1 : Selector  InputPortWidth=4  IndexOptions=Index vector (dialog)  Indices=[3:4]  OutputSizes=1
  Subsystem : Subsystem
  Subsystem1 : Subsystem
  rd_dout1 : Outport  PortDimensions=4  VectorParamsAs1DForOutWhenUnconnected=off
  wires:
  rd_addr1/1 -> Subsystem1/4(rd_addr), Subsystem/4(rd_addr)
  Mux1/1 -> rd_dout1/1
  data2/1 -> Selector/1, Selector1/1
  wr_en2/1 -> Subsystem1/3(wr_en), Subsystem/3(wr_en)
  Selector1/1 -> Subsystem1/1(data)
  wr_addr1/1 -> Subsystem1/2(wr_addr), Subsystem/2(wr_addr)
  Subsystem1/1(rd_dout) -> Mux1/2
  Subsystem/1(rd_dout) -> Mux1/1
  Selector/1 -> Subsystem/1(data)

== system rx2/process5/decoder/p-p/Subsystem2/Subsystem/Subsystem2/Subsystem/Subsystem4 ==
  data2 : Inport  OutDataTypeStr=data_type
  wr_addr1 : Inport  Port=2
  wr_en2 : Inport  Port=3
  rd_addr1 : Inport  Port=4
  Mux1 : Mux  Inputs=2
  Selector : Selector  InputPortWidth=4  IndexOptions=Index vector (dialog)  Indices=[1:2]  OutputSizes=1
  Selector1 : Selector  InputPortWidth=4  IndexOptions=Index vector (dialog)  Indices=[3:4]  OutputSizes=1
  Subsystem : Subsystem
  Subsystem1 : Subsystem
  rd_dout1 : Outport  PortDimensions=4  VectorParamsAs1DForOutWhenUnconnected=off
  wires:
  Selector/1 -> Subsystem/1(data)
  Subsystem/1(rd_dout) -> Mux1/1
  Subsystem1/1(rd_dout) -> Mux1/2
  wr_addr1/1 -> Subsystem/2(wr_addr), Subsystem1/2(wr_addr)
  Selector1/1 -> Subsystem1/1(data)
  wr_en2/1 -> Subsystem/3(wr_en), Subsystem1/3(wr_en)
  data2/1 -> Selector1/1, Selector/1
  Mux1/1 -> rd_dout1/1
  rd_addr1/1 -> Subsystem/4(rd_addr), Subsystem1/4(rd_addr)

== system rx2/process5/decoder/p-p/Subsystem2/Subsystem/Subsystem2/Subsystem1/Subsystem1 ==
  data2 : Inport  OutDataTypeStr=data_type
  wr_addr1 : Inport  Port=2
  wr_en2 : Inport  Port=3
  rd_addr1 : Inport  Port=4
  Mux1 : Mux  Inputs=2
  Selector : Selector  InputPortWidth=4  IndexOptions=Index vector (dialog)  Indices=[1:2]  OutputSizes=1
  Selector1 : Selector  InputPortWidth=4  IndexOptions=Index vector (dialog)  Indices=[3:4]  OutputSizes=1
  Subsystem : Subsystem
  Subsystem1 : Subsystem
  rd_dout1 : Outport  PortDimensions=4  VectorParamsAs1DForOutWhenUnconnected=off
  wires:
  rd_addr1/1 -> Subsystem1/4(rd_addr), Subsystem/4(rd_addr)
  Mux1/1 -> rd_dout1/1
  data2/1 -> Selector/1, Selector1/1
  wr_en2/1 -> Subsystem1/3(wr_en), Subsystem/3(wr_en)
  Selector1/1 -> Subsystem1/1(data)
  wr_addr1/1 -> Subsystem1/2(wr_addr), Subsystem/2(wr_addr)
  Subsystem1/1(rd_dout) -> Mux1/2
  Subsystem/1(rd_dout) -> Mux1/1
  Selector/1 -> Subsystem/1(data)

== system rx2/process5/decoder/p-p/Subsystem2/Subsystem/Subsystem2/Subsystem1/Subsystem4 ==
  data2 : Inport  OutDataTypeStr=data_type
  wr_addr1 : Inport  Port=2
  wr_en2 : Inport  Port=3
  rd_addr1 : Inport  Port=4
  Mux1 : Mux  Inputs=2
  Selector : Selector  InputPortWidth=4  IndexOptions=Index vector (dialog)  Indices=[1:2]  OutputSizes=1
  Selector1 : Selector  InputPortWidth=4  IndexOptions=Index vector (dialog)  Indices=[3:4]  OutputSizes=1
  Subsystem : Subsystem
  Subsystem1 : Subsystem
  rd_dout1 : Outport  PortDimensions=4  VectorParamsAs1DForOutWhenUnconnected=off
  wires:
  rd_addr1/1 -> Subsystem1/4(rd_addr), Subsystem/4(rd_addr)
  Mux1/1 -> rd_dout1/1
  data2/1 -> Selector/1, Selector1/1
  wr_en2/1 -> Subsystem1/3(wr_en), Subsystem/3(wr_en)
  Selector1/1 -> Subsystem1/1(data)
  wr_addr1/1 -> Subsystem1/2(wr_addr), Subsystem/2(wr_addr)
  Subsystem1/1(rd_dout) -> Mux1/2
  Subsystem/1(rd_dout) -> Mux1/1
  Selector/1 -> Subsystem/1(data)

== system rx2/process5/decoder/p-p/Subsystem2/Subsystem1/Subsystem1/Subsystem/Subsystem1 ==
  data2 : Inport  OutDataTypeStr=data_type
  wr_addr1 : Inport  Port=2
  wr_en2 : Inport  Port=3
  rd_addr1 : Inport  Port=4
  Mux1 : Mux  Inputs=2
  Selector : Selector  InputPortWidth=4  IndexOptions=Index vector (dialog)  Indices=[1:2]  OutputSizes=1
  Selector1 : Selector  InputPortWidth=4  IndexOptions=Index vector (dialog)  Indices=[3:4]  OutputSizes=1
  Subsystem : Subsystem
  Subsystem1 : Subsystem
  rd_dout1 : Outport  PortDimensions=4  VectorParamsAs1DForOutWhenUnconnected=off
  wires:
  rd_addr1/1 -> Subsystem1/4(rd_addr), Subsystem/4(rd_addr)
  Mux1/1 -> rd_dout1/1
  data2/1 -> Selector/1, Selector1/1
  wr_en2/1 -> Subsystem1/3(wr_en), Subsystem/3(wr_en)
  Selector1/1 -> Subsystem1/1(data)
  wr_addr1/1 -> Subsystem1/2(wr_addr), Subsystem/2(wr_addr)
  Subsystem1/1(rd_dout) -> Mux1/2
  Subsystem/1(rd_dout) -> Mux1/1
  Selector/1 -> Subsystem/1(data)

== system rx2/process5/decoder/p-p/Subsystem2/Subsystem1/Subsystem1/Subsystem/Subsystem4 ==
  data2 : Inport  OutDataTypeStr=data_type
  wr_addr1 : Inport  Port=2
  wr_en2 : Inport  Port=3
  rd_addr1 : Inport  Port=4
  Mux1 : Mux  Inputs=2
  Selector : Selector  InputPortWidth=4  IndexOptions=Index vector (dialog)  Indices=[1:2]  OutputSizes=1
  Selector1 : Selector  InputPortWidth=4  IndexOptions=Index vector (dialog)  Indices=[3:4]  OutputSizes=1
  Subsystem : Subsystem
  Subsystem1 : Subsystem
  rd_dout1 : Outport  PortDimensions=4  VectorParamsAs1DForOutWhenUnconnected=off
  wires:
  Selector/1 -> Subsystem/1(data)
  Subsystem/1(rd_dout) -> Mux1/1
  Subsystem1/1(rd_dout) -> Mux1/2
  wr_addr1/1 -> Subsystem/2(wr_addr), Subsystem1/2(wr_addr)
  Selector1/1 -> Subsystem1/1(data)
  wr_en2/1 -> Subsystem/3(wr_en), Subsystem1/3(wr_en)
  data2/1 -> Selector1/1, Selector/1
  Mux1/1 -> rd_dout1/1
  rd_addr1/1 -> Subsystem/4(rd_addr), Subsystem1/4(rd_addr)

== system rx2/process5/decoder/p-p/Subsystem2/Subsystem1/Subsystem1/Subsystem1/Subsystem1 ==
  data2 : Inport  OutDataTypeStr=data_type
  wr_addr1 : Inport  Port=2
  wr_en2 : Inport  Port=3
  rd_addr1 : Inport  Port=4
  Mux1 : Mux  Inputs=2
  Selector : Selector  InputPortWidth=4  IndexOptions=Index vector (dialog)  Indices=[1:2]  OutputSizes=1
  Selector1 : Selector  InputPortWidth=4  IndexOptions=Index vector (dialog)  Indices=[3:4]  OutputSizes=1
  Subsystem : Subsystem
  Subsystem1 : Subsystem
  rd_dout1 : Outport  PortDimensions=4  VectorParamsAs1DForOutWhenUnconnected=off
  wires:
  rd_addr1/1 -> Subsystem1/4(rd_addr), Subsystem/4(rd_addr)
  Mux1/1 -> rd_dout1/1
  data2/1 -> Selector/1, Selector1/1
  wr_en2/1 -> Subsystem1/3(wr_en), Subsystem/3(wr_en)
  Selector1/1 -> Subsystem1/1(data)
  wr_addr1/1 -> Subsystem1/2(wr_addr), Subsystem/2(wr_addr)
  Subsystem1/1(rd_dout) -> Mux1/2
  Subsystem/1(rd_dout) -> Mux1/1
  Selector/1 -> Subsystem/1(data)

== system rx2/process5/decoder/p-p/Subsystem2/Subsystem1/Subsystem1/Subsystem1/Subsystem4 ==
  data2 : Inport  OutDataTypeStr=data_type
  wr_addr1 : Inport  Port=2
  wr_en2 : Inport  Port=3
  rd_addr1 : Inport  Port=4
  Mux1 : Mux  Inputs=2
  Selector : Selector  InputPortWidth=4  IndexOptions=Index vector (dialog)  Indices=[1:2]  OutputSizes=1
  Selector1 : Selector  InputPortWidth=4  IndexOptions=Index vector (dialog)  Indices=[3:4]  OutputSizes=1
  Subsystem : Subsystem
  Subsystem1 : Subsystem
  rd_dout1 : Outport  PortDimensions=4  VectorParamsAs1DForOutWhenUnconnected=off
  wires:
  rd_addr1/1 -> Subsystem1/4(rd_addr), Subsystem/4(rd_addr)
  Mux1/1 -> rd_dout1/1
  data2/1 -> Selector/1, Selector1/1
  wr_en2/1 -> Subsystem1/3(wr_en), Subsystem/3(wr_en)
  Selector1/1 -> Subsystem1/1(data)
  wr_addr1/1 -> Subsystem1/2(wr_addr), Subsystem/2(wr_addr)
  Subsystem1/1(rd_dout) -> Mux1/2
  Subsystem/1(rd_dout) -> Mux1/1
  Selector/1 -> Subsystem/1(data)

== system rx2/process5/decoder/p-p/Subsystem2/Subsystem1/Subsystem2/Subsystem/Subsystem1 ==
  data2 : Inport  OutDataTypeStr=data_type
  wr_addr1 : Inport  Port=2
  wr_en2 : Inport  Port=3
  rd_addr1 : Inport  Port=4
  Mux1 : Mux  Inputs=2
  Selector : Selector  InputPortWidth=4  IndexOptions=Index vector (dialog)  Indices=[1:2]  OutputSizes=1
  Selector1 : Selector  InputPortWidth=4  IndexOptions=Index vector (dialog)  Indices=[3:4]  OutputSizes=1
  Subsystem : Subsystem
  Subsystem1 : Subsystem
  rd_dout1 : Outport  PortDimensions=4  VectorParamsAs1DForOutWhenUnconnected=off
  wires:
  rd_addr1/1 -> Subsystem1/4(rd_addr), Subsystem/4(rd_addr)
  Mux1/1 -> rd_dout1/1
  data2/1 -> Selector/1, Selector1/1
  wr_en2/1 -> Subsystem1/3(wr_en), Subsystem/3(wr_en)
  Selector1/1 -> Subsystem1/1(data)
  wr_addr1/1 -> Subsystem1/2(wr_addr), Subsystem/2(wr_addr)
  Subsystem1/1(rd_dout) -> Mux1/2
  Subsystem/1(rd_dout) -> Mux1/1
  Selector/1 -> Subsystem/1(data)

== system rx2/process5/decoder/p-p/Subsystem2/Subsystem1/Subsystem2/Subsystem/Subsystem4 ==
  data2 : Inport  OutDataTypeStr=data_type
  wr_addr1 : Inport  Port=2
  wr_en2 : Inport  Port=3
  rd_addr1 : Inport  Port=4
  Mux1 : Mux  Inputs=2
  Selector : Selector  InputPortWidth=4  IndexOptions=Index vector (dialog)  Indices=[1:2]  OutputSizes=1
  Selector1 : Selector  InputPortWidth=4  IndexOptions=Index vector (dialog)  Indices=[3:4]  OutputSizes=1
  Subsystem : Subsystem
  Subsystem1 : Subsystem
  rd_dout1 : Outport  PortDimensions=4  VectorParamsAs1DForOutWhenUnconnected=off
  wires:
  Selector/1 -> Subsystem/1(data)
  Subsystem/1(rd_dout) -> Mux1/1
  Subsystem1/1(rd_dout) -> Mux1/2
  wr_addr1/1 -> Subsystem/2(wr_addr), Subsystem1/2(wr_addr)
  Selector1/1 -> Subsystem1/1(data)
  wr_en2/1 -> Subsystem/3(wr_en), Subsystem1/3(wr_en)
  data2/1 -> Selector1/1, Selector/1
  Mux1/1 -> rd_dout1/1
  rd_addr1/1 -> Subsystem/4(rd_addr), Subsystem1/4(rd_addr)

== system rx2/process5/decoder/p-p/Subsystem2/Subsystem1/Subsystem2/Subsystem1/Subsystem1 ==
  data2 : Inport  OutDataTypeStr=data_type
  wr_addr1 : Inport  Port=2
  wr_en2 : Inport  Port=3
  rd_addr1 : Inport  Port=4
  Mux1 : Mux  Inputs=2
  Selector : Selector  InputPortWidth=4  IndexOptions=Index vector (dialog)  Indices=[1:2]  OutputSizes=1
  Selector1 : Selector  InputPortWidth=4  IndexOptions=Index vector (dialog)  Indices=[3:4]  OutputSizes=1
  Subsystem : Subsystem
  Subsystem1 : Subsystem
  rd_dout1 : Outport  PortDimensions=4  VectorParamsAs1DForOutWhenUnconnected=off
  wires:
  rd_addr1/1 -> Subsystem1/4(rd_addr), Subsystem/4(rd_addr)
  Mux1/1 -> rd_dout1/1
  data2/1 -> Selector/1, Selector1/1
  wr_en2/1 -> Subsystem1/3(wr_en), Subsystem/3(wr_en)
  Selector1/1 -> Subsystem1/1(data)
  wr_addr1/1 -> Subsystem1/2(wr_addr), Subsystem/2(wr_addr)
  Subsystem1/1(rd_dout) -> Mux1/2
  Subsystem/1(rd_dout) -> Mux1/1
  Selector/1 -> Subsystem/1(data)

== system rx2/process5/decoder/p-p/Subsystem2/Subsystem1/Subsystem2/Subsystem1/Subsystem4 ==
  data2 : Inport  OutDataTypeStr=data_type
  wr_addr1 : Inport  Port=2
  wr_en2 : Inport  Port=3
  rd_addr1 : Inport  Port=4
  Mux1 : Mux  Inputs=2
  Selector : Selector  InputPortWidth=4  IndexOptions=Index vector (dialog)  Indices=[1:2]  OutputSizes=1
  Selector1 : Selector  InputPortWidth=4  IndexOptions=Index vector (dialog)  Indices=[3:4]  OutputSizes=1
  Subsystem : Subsystem
  Subsystem1 : Subsystem
  rd_dout1 : Outport  PortDimensions=4  VectorParamsAs1DForOutWhenUnconnected=off
  wires:
  rd_addr1/1 -> Subsystem1/4(rd_addr), Subsystem/4(rd_addr)
  Mux1/1 -> rd_dout1/1
  data2/1 -> Selector/1, Selector1/1
  wr_en2/1 -> Subsystem1/3(wr_en), Subsystem/3(wr_en)
  Selector1/1 -> Subsystem1/1(data)
  wr_addr1/1 -> Subsystem1/2(wr_addr), Subsystem/2(wr_addr)
  Subsystem1/1(rd_dout) -> Mux1/2
  Subsystem/1(rd_dout) -> Mux1/1
  Selector/1 -> Subsystem/1(data)

== system rx2/process6/decoder/p-p/Subsystem2/Subsystem/Subsystem1/Subsystem/Subsystem1 ==
  data2 : Inport  OutDataTypeStr=data_type
  wr_addr1 : Inport  Port=2
  wr_en2 : Inport  Port=3
  rd_addr1 : Inport  Port=4
  Mux1 : Mux  Inputs=2
  Selector : Selector  InputPortWidth=4  IndexOptions=Index vector (dialog)  Indices=[1:2]  OutputSizes=1
  Selector1 : Selector  InputPortWidth=4  IndexOptions=Index vector (dialog)  Indices=[3:4]  OutputSizes=1
  Subsystem : Subsystem
  Subsystem1 : Subsystem
  rd_dout1 : Outport  PortDimensions=4  VectorParamsAs1DForOutWhenUnconnected=off
  wires:
  Selector/1 -> Subsystem/1(data)
  Subsystem/1(rd_dout) -> Mux1/1
  Subsystem1/1(rd_dout) -> Mux1/2
  wr_addr1/1 -> Subsystem/2(wr_addr), Subsystem1/2(wr_addr)
  Selector1/1 -> Subsystem1/1(data)
  wr_en2/1 -> Subsystem/3(wr_en), Subsystem1/3(wr_en)
  data2/1 -> Selector1/1, Selector/1
  Mux1/1 -> rd_dout1/1
  rd_addr1/1 -> Subsystem/4(rd_addr), Subsystem1/4(rd_addr)

== system rx2/process6/decoder/p-p/Subsystem2/Subsystem/Subsystem1/Subsystem/Subsystem4 ==
  data2 : Inport  OutDataTypeStr=data_type
  wr_addr1 : Inport  Port=2
  wr_en2 : Inport  Port=3
  rd_addr1 : Inport  Port=4
  Mux1 : Mux  Inputs=2
  Selector : Selector  InputPortWidth=4  IndexOptions=Index vector (dialog)  Indices=[1:2]  OutputSizes=1
  Selector1 : Selector  InputPortWidth=4  IndexOptions=Index vector (dialog)  Indices=[3:4]  OutputSizes=1
  Subsystem : Subsystem
  Subsystem1 : Subsystem
  rd_dout1 : Outport  PortDimensions=4  VectorParamsAs1DForOutWhenUnconnected=off
  wires:
  rd_addr1/1 -> Subsystem1/4(rd_addr), Subsystem/4(rd_addr)
  Mux1/1 -> rd_dout1/1
  data2/1 -> Selector/1, Selector1/1
  wr_en2/1 -> Subsystem1/3(wr_en), Subsystem/3(wr_en)
  Selector1/1 -> Subsystem1/1(data)
  wr_addr1/1 -> Subsystem1/2(wr_addr), Subsystem/2(wr_addr)
  Subsystem1/1(rd_dout) -> Mux1/2
  Subsystem/1(rd_dout) -> Mux1/1
  Selector/1 -> Subsystem/1(data)

== system rx2/process6/decoder/p-p/Subsystem2/Subsystem/Subsystem1/Subsystem1/Subsystem1 ==
  data2 : Inport  OutDataTypeStr=data_type
  wr_addr1 : Inport  Port=2
  wr_en2 : Inport  Port=3
  rd_addr1 : Inport  Port=4
  Mux1 : Mux  Inputs=2
  Selector : Selector  InputPortWidth=4  IndexOptions=Index vector (dialog)  Indices=[1:2]  OutputSizes=1
  Selector1 : Selector  InputPortWidth=4  IndexOptions=Index vector (dialog)  Indices=[3:4]  OutputSizes=1
  Subsystem : Subsystem
  Subsystem1 : Subsystem
  rd_dout1 : Outport  PortDimensions=4  VectorParamsAs1DForOutWhenUnconnected=off
  wires:
  Selector/1 -> Subsystem/1(data)
  Subsystem/1(rd_dout) -> Mux1/1
  Subsystem1/1(rd_dout) -> Mux1/2
  wr_addr1/1 -> Subsystem/2(wr_addr), Subsystem1/2(wr_addr)
  Selector1/1 -> Subsystem1/1(data)
  wr_en2/1 -> Subsystem/3(wr_en), Subsystem1/3(wr_en)
  data2/1 -> Selector1/1, Selector/1
  Mux1/1 -> rd_dout1/1
  rd_addr1/1 -> Subsystem/4(rd_addr), Subsystem1/4(rd_addr)

== system rx2/process6/decoder/p-p/Subsystem2/Subsystem/Subsystem1/Subsystem1/Subsystem4 ==
  data2 : Inport  OutDataTypeStr=data_type
  wr_addr1 : Inport  Port=2
  wr_en2 : Inport  Port=3
  rd_addr1 : Inport  Port=4
  Mux1 : Mux  Inputs=2
  Selector : Selector  InputPortWidth=4  IndexOptions=Index vector (dialog)  Indices=[1:2]  OutputSizes=1
  Selector1 : Selector  InputPortWidth=4  IndexOptions=Index vector (dialog)  Indices=[3:4]  OutputSizes=1
  Subsystem : Subsystem
  Subsystem1 : Subsystem
  rd_dout1 : Outport  PortDimensions=4  VectorParamsAs1DForOutWhenUnconnected=off
  wires:
  Selector/1 -> Subsystem/1(data)
  Subsystem/1(rd_dout) -> Mux1/1
  Subsystem1/1(rd_dout) -> Mux1/2
  wr_addr1/1 -> Subsystem/2(wr_addr), Subsystem1/2(wr_addr)
  Selector1/1 -> Subsystem1/1(data)
  wr_en2/1 -> Subsystem/3(wr_en), Subsystem1/3(wr_en)
  data2/1 -> Selector1/1, Selector/1
  Mux1/1 -> rd_dout1/1
  rd_addr1/1 -> Subsystem/4(rd_addr), Subsystem1/4(rd_addr)
